simulink subsystem "SolarPressure_SS"  (R2023a)
settings: Solver=VariableStepAuto  StartTime=0.0  StopTime=10.0  RelTol=1e-3
undefined symbols (not defined in the file or in its folder): srp
settings Model: Creator=jself  LastModifiedBy=shaniyasingh

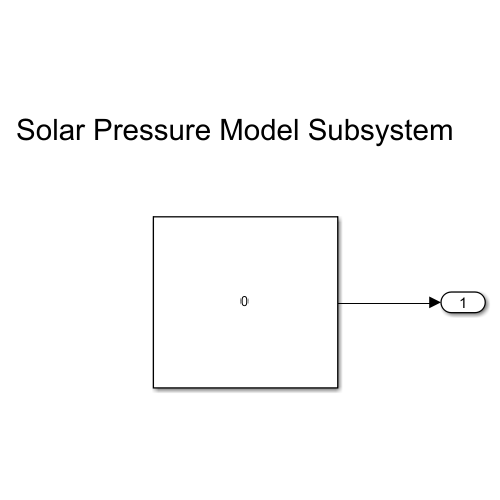
[thumbnail: Simulink's stored preview of the top-level diagram]
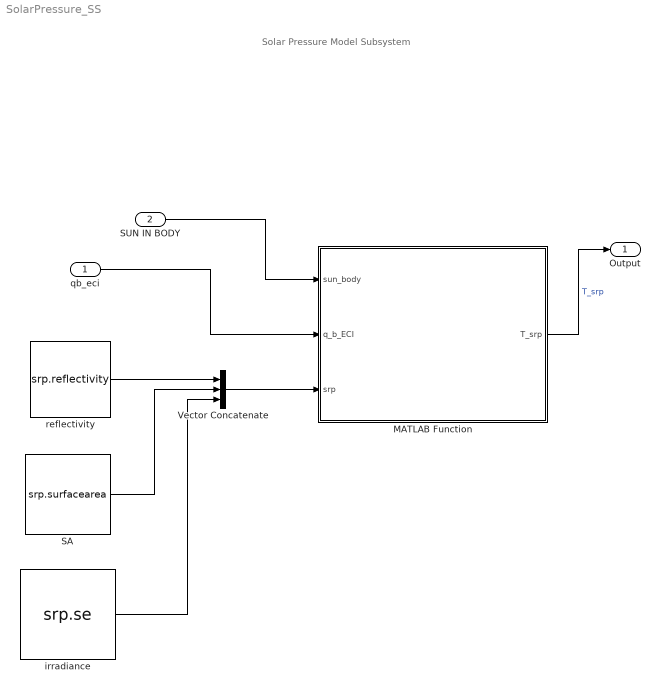
== system SolarPressure_SS ==
  note: Solar Pressure Model Subsystem
  qb_eci : Inport
  SUN IN BODY : Inport  Port=2
  MATLAB Function : MATLAB Function  TreatAsAtomicUnit=on
  SA : Constant  Value=srp.surfacearea
  Vector Concatenate : Concatenate  NumInputs=3
  irradiance : Constant  Value=srp.se
  reflectivity : Constant  Value=srp.reflectivity
  Output : Outport
  wires:
  MATLAB Function/1(T_srp) -> Output/1  "T_srp"
  reflectivity/1 -> Vector Concatenate/1
  SA/1 -> Vector Concatenate/2
  Vector Concatenate/1 -> MATLAB Function/3(srp)
  irradiance/1 -> Vector Concatenate/3
  qb_eci/1 -> MATLAB Function/2(q_b_ECI)
  SUN IN BODY/1 -> MATLAB Function/1(sun_body)

== matlab function SolarPressure_SS/MATLAB Function ==
  data: sun_body input; T_srp output; q_b_ECI input; srp input
function T_srp  = SRP_torque(sun_body, q_b_ECI, srp)

% Calculate solar radiation pressure torque
% Note this is not using lecture notes to avoid center of pressure calcs :)
% Jk it is to match Mehiel's ugly code where he did not even use his own
% notes.

% NOTE: quaternion is [eta;epsilonx;epsilony; epsilonz];
% NOPE: its actually [epsilon; eta]

% surface properties == 1. reflec; 2. S_area 3. solar irradiance
% Constants
c = 2.998e8; % Speed of light in m/s

% Surface properties
A = srp(2);
reflectivity = srp(1);
irradiance = srp(3);

% Relative velocity 

v_rel_ECI = -cross(sun_body, q_b_ECI(1:3));
v_rel_mag = norm(v_rel_ECI);

% Solar radiation pressure
P_srp = c * irradiance / (4 * reflectivity);
%P_srp = irradiance/c;
% P_srp = (irradiance*(reflectivity+1))/c;
% P_srp = 4.5e-6;
% conversion = 1/(1000^6);
conversion = 1;
% Solar radiation pressure torque
T_srp = conversion * -P_srp * A * v_rel_mag * cross(v_rel_ECI, q_b_ECI(1:3));

% Total accumulated solar radiation pressure
rho_sum = P_srp * A;

end
